simulink model "lab_04_simulink_conflict_copy_DESKTOP-NCVGOGC_2025_04_12"  (R2024b)
settings: Solver=VariableStepAuto  StartTime=0.0  StopTime=10.0  RelTol=1e-3
settings Model: LastModifiedBy=LENOVO
settings RTWCC: GenCodeOnly=on

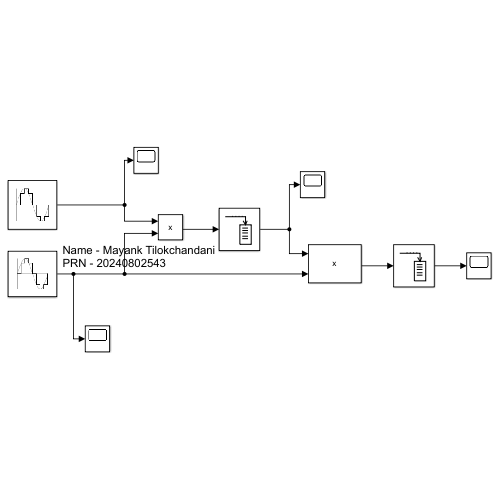
[thumbnail: Simulink's stored preview of the top-level diagram]
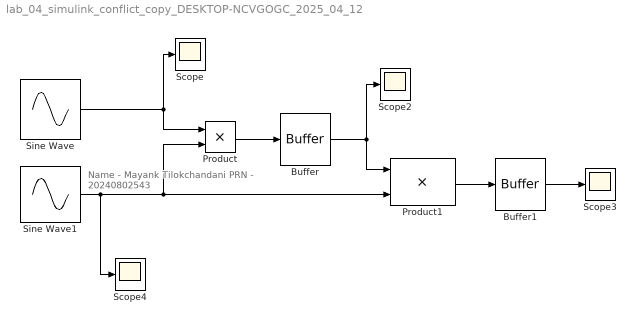
== system lab_04_simulink_conflict_copy_DESKTOP-NCVGOGC_2025_04_12 ==
  note: Name - Mayank Tilokchandani
      | PRN - 20240802543
  Buffer : Buffer  N=1  OutputFrames=off
  Buffer1 : Buffer  N=1  OutputFrames=off
  Product : Product
  Product1 : Product
  Scope{,2..4} (4 alike) : Scope
  Sine Wave : Sin  Amplitude=2  SampleTime=0.01
  Sine Wave1 : Sin  Amplitude=2  Frequency=10  SampleTime=0.01
  wires:
  Sine Wave/1 -> Scope/1, Product/1
  Sine Wave1/1 -> Scope4/1, Product1/2, Product/2
  Product/1 -> Buffer/1
  Buffer/1 -> Scope2/1, Product1/1
  Product1/1 -> Buffer1/1
  Buffer1/1 -> Scope3/1
